simulink library "convolution"  (R2015b)
settings: Solver=VariableStepAuto  StartTime=0.0  StopTime=10.0  RelTol=1e-3
values from neighbouring files (symbols this model uses):
  dt = 0.00005    (= 5e-05)    [param.m]
undefined symbols (not defined in the file or in its folder): DiscIntNeverNeededParam
settings Model: Creator=mishuk  LastModifiedBy=mishuk

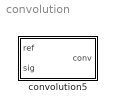
== system convolution ==
  convolution5 : Subsystem  mask(Convolution){delay=1000}
      mask prompts: delay "Reference delay"
      mask help: Convolution of signal & reference inputs

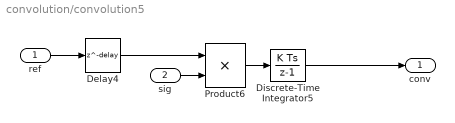
== system convolution/convolution5 ==
  ref : Inport
  sig : Inport  Port=2
  Delay4 : Delay  DelayLength=delay
  Discrete-Time Integrator5 : DiscreteIntegrator  SampleTime=dt  ICPrevOutput=DiscIntNeverNeededParam  ICPrevScaledInput=DiscIntNeverNeededParam
  Product6 : Product  RndMeth=Zero
  conv : Outport
  wires:
  Discrete-Time Integrator5/1 -> conv/1
  ref/1 -> Delay4/1
  Product6/1 -> Discrete-Time Integrator5/1
  sig/1 -> Product6/2
  Delay4/1 -> Product6/1
